simulink model "rtwdemo_sil_hardware_config"  (Simulink 7.6)
settings: Solver=ode3  StartTime=0.0  StopTime=20  FixedStep=0.01  RelTol=1e-3
libraries: rtwdemowidgets x2
Description:
  | Hardware Configuration Options for Software-in-the-Loop Verification
CloseFcn:
  | rtwprivate ssgencode ModelCloseRequest rtwdemo_sil_hardware_config
settings Model: Creator=The MathWorks Inc.  ExtModeAutoUpdateStatusClock=off
settings MATStruct: SampleTime=0.01  Offset=0  Priority=[20.0]
settings DataIOCC: SaveOutput=off  SaveTime=off  SignalLoggingName=sigsOut
settings OptimizationCC: InlineParams=on  InlineInvariantSignals=on  PassReuseOutputArgsAs=Individual arguments  StateBitsets=on  DataBitsets=on  UseTempVars=on  ZeroExternalMemoryAtStartup=off  ZeroInternalMemoryAtStartup=off  NoFixptDivByZeroProtection=on  EfficientFloat2IntCast=on  EfficientMapNaN2IntZero=off  OptimizeModelRefInitCode=on  LifeSpan=1
settings DebuggingCC: UnderspecifiedInitializationDetection=Simplified  MergeDetectMultiDrivingBlocksExec=error  CheckExecutionContextPreStartOutputMsg=on  CheckExecutionContextRuntimeOutputMsg=on  SolverPrmCheckMsg=none  StrictBusMsg=ErrorOnBusTreatedAsVector
settings HardwareCC: ProdBitPerInt=16  ProdIntDivRoundTo=Zero  ProdEndianess=LittleEndian  ProdWordSize=16  ProdHWDeviceType=Generic->16-bit Embedded Processor  TargetEndianess=LittleEndian  TargetHWDeviceType=Generic->MATLAB Host Computer  ProdEqTarget=off
settings RTWCC: SystemTargetFile=ert.tlc  TemplateMakefile=ert_default_tmf  GenerateReport=on  RTWVerbose=off  ProcessScript=ert_make_rtw_hook  IncludeHyperlinkInReport=on  LaunchReport=on
settings CodeAppCC: ForceParamTrailComments=on  IgnoreCustomStorageClasses=off  IgnoreTestpoints=on  SimulinkDataObjDesc=on  CustomSymbolStrGlobalVar=rt$N$M  CustomSymbolStrType=$N$M  CustomSymbolStrFcn=$N$M$F  CustomSymbolStrMacro=$N$M  InsertBlockDesc=on
settings ERTTargetCC: TargetFcnLib=ansi_tfl_tmw.mat  MultiwordLength=2048  GenerateSampleERTMain=on  IncludeMdlTerminateFcn=off  SupportNonFinite=off  SupportComplex=off  SupportContinuousTime=on  GenerateErtSFunction=on  CreateSILPILBlock=SIL  InlinedParameterPlacement=NonHierarchical  ERTCustomFileTemplate=example_file_process.tlc  ERTFilePackagingFormat=CompactWithDataFile  ConvertIfToSwitch=off

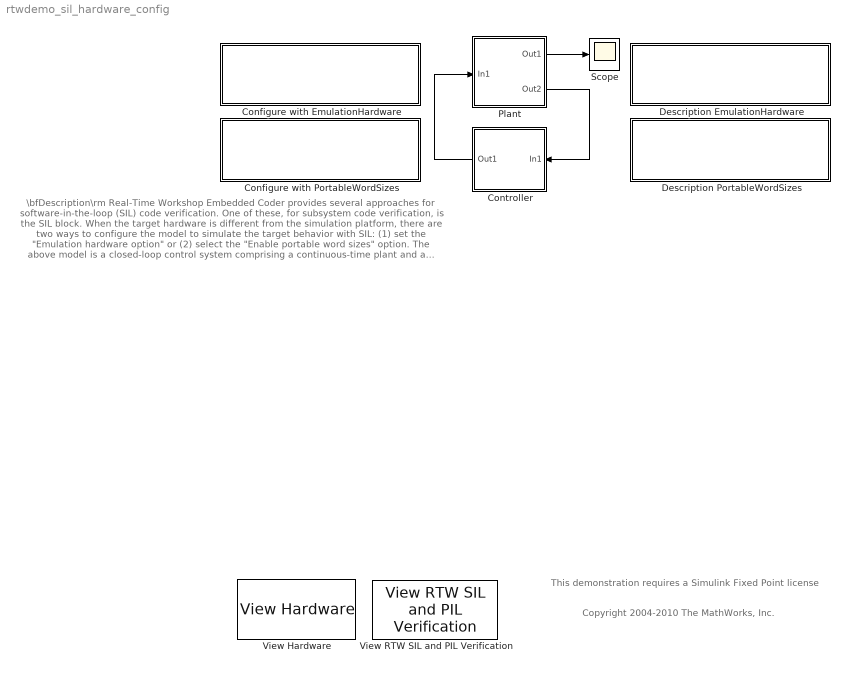
== system rtwdemo_sil_hardware_config ==
  note: \bfDescription\rm
      | Real-Time Workshop Embedded Coder provides several approaches for software-in-the-loop (SIL)
      | code verification. One of these, for subsystem code verification, is the SIL block.
      | When the target hardware is different from the simulation platform, there are two ways to configure
      | the model to simulate the target behavior with SIL: (1) set the "Emulation hardware option" or
      | (2) select the "Enable portable word sizes" option. The above model is a closed-loop control
      | system comprising a continuous-time plant and a discrete-time controller to be deployed on a
      | generic 16-bit microcontroller. The Controller subsystem employs fixed-point arithmetic. An
      | overflow effect is intentionally added to help compare simulation results. To read more about
      | each option, click the above grey buttons. Click the yellow buttons to view the configuration panels.
      |
      | \bfInstructions\rm
      | 1. Click either of the blue buttons above to configure the model automatically.
      | 2. Right-click the Controller subsystem and select Real-Time Workshop > Build Subsystem.
      | 3. When the parameter dialog appears, click the Build button. The SIL block is created in
      |     an untitled model.  This SIL block is an S-function wrapper for the generated subsystem code,
      |     and can be used to verify that the code provides the same result as the original subsystem.
      | 4. Replace the original system with the S-function block and rerun the simulation to verify that the
      |     output is correct. Observe the overflow effect at around 10.8 seconds.
  note: Copyright 2004-2010 The MathWorks, Inc.
  note: This demonstration requires a Simulink Fixed Point license
  Configure with EmulationHardware : Subsystem
      settings: OpenFcn=|
      | try
      |   set_param(gcs, 'GenerateErtSFunction', 'on');
      |   set_param(gcs, 'ProdEqTarget','off');            set_param(gcs, 'PortableWordSizes','off');
      |   set_param(gcs, 'TargetHWDeviceType', 'MATLAB Host');
      | catch
      |   disp('cannot auto configure.');
      |   rethrow(lasterror);
      | end
      mask Type: Auto Config
      mask Display: disp(['Configure with \nEmulation Hardware Setup\n(double-click)'])
  Configure with PortableWordSizes : Subsystem
      settings: OpenFcn=|
      | try
      |   set_param(gcs, 'GenerateErtSFunction', 'on');
      |   set_param(gcs, 'ProdEqTarget','on');             set_param(gcs, 'PortableWordSizes','on');
      | catch
      |     error('cannot auto configure.');
      | end
      mask Display: disp(['Configure with \nPortable Word Sizes Setup\n(double-click)'])
  Controller : Subsystem  TreatAsAtomicUnit=on
      settings: RTWFcnNameOpts=Use subsystem name  RTWFileNameOpts=Use function name
  Description EmulationHardware : Subsystem
      mask Display: disp(['View Description of\n Emulation Hardware Setup\n(double-click)'])
  Description PortableWordSizes : Subsystem
      mask Display: disp(['View Description of \nPortable Word Sizes Setup\n(double-click)'])
  Plant : Subsystem
  Scope : Scope
      settings: TimeRange=20  YMin=0  YMax=400
  View Hardware : rtwdemowidgets/View Hardware  SystemSampleTime=-1
  View RTW SIL and PIL Verification : rtwdemowidgets/View RTW SIL and PIL Verification  SystemSampleTime=-1
  wires:
  Plant/1(Out1) -> Scope/1
  Plant/2(Out2) -> Controller/1(In1)
  Controller/1(Out1) -> Plant/1(In1)

== system rtwdemo_sil_hardware_config/Configure with EmulationHardware ==

== system rtwdemo_sil_hardware_config/Configure with PortableWordSizes ==

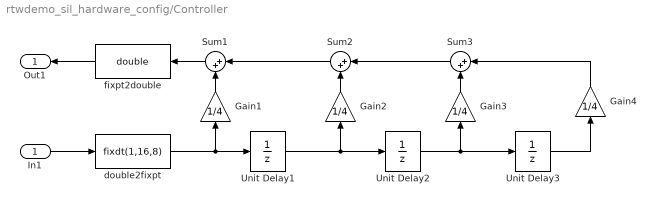
== system rtwdemo_sil_hardware_config/Controller ==
  In1 : Inport  SampleTime=.01
  Gain{1..4} (4 alike) : Gain  Gain=1/4  SaturateOnIntegerOverflow=on  ParamDataTypeStr=Inherit: Same as input
  Sum1 : Sum  Inputs=|++  SaturateOnIntegerOverflow=on  InputSameDT=on  OutDataTypeStr=Inherit: Same as first input
  Sum2 : Sum  Inputs=|++  SaturateOnIntegerOverflow=on  InputSameDT=on  OutDataTypeStr=Inherit: Same as first input
  Sum3 : Sum  Inputs=|++  SaturateOnIntegerOverflow=on  InputSameDT=on  OutDataTypeStr=Inherit: Same as first input
  Unit Delay1 : UnitDelay  SampleTime=-1
  Unit Delay2 : UnitDelay  SampleTime=-1
  Unit Delay3 : UnitDelay  SampleTime=-1
  double2fixpt : DataTypeConversion  OutDataTypeStr=fixdt(1,16,8)
  fixpt2double : DataTypeConversion  OutDataTypeStr=double
  Out1 : Outport
  wires:
  Gain1/1 -> Sum1/2
  In1/1 -> double2fixpt/1
  Sum1/1 -> fixpt2double/1
  Sum3/1 -> Sum2/1
  Sum2/1 -> Sum1/1
  Unit Delay1/1 -> Unit Delay2/1, Gain2/1
  Unit Delay2/1 -> Unit Delay3/1, Gain3/1
  Unit Delay3/1 -> Gain4/1
  Gain4/1 -> Sum3/1
  Gain3/1 -> Sum3/2
  Gain2/1 -> Sum2/2
  double2fixpt/1 -> Unit Delay1/1, Gain1/1
  fixpt2double/1 -> Out1/1

== system rtwdemo_sil_hardware_config/Description EmulationHardware ==
  note: \bfDescription\rm
      | You may need to use the host platform to simulate the exact behavior of the generated code on the
      | embedded system where it will be deployed. Choose to create a SIL block with
      | the emulation hardware set to the host platform.  In this case, Real-Time Workshop inserts any additional
      | code (e.g., data type casts) that is necessary to ensure behavior consistent with the target environment.
      | After the simulation, choose "None" for emulation hardware and regenerate the code before deployment.
      |
      | \bfManual Configuration\rm
      | 1. Open the Hardware Implementation page by double-clicking the first yellow button at the bottom. Select
      |     "MATLAB Host Computer" as Emulation hardware.
      | 2. Open the Real-Time Workshop SIL and PIL Verification page by double-clicking the second yellow
      |      button at the bottom. Ensure that the "Create block" option is set to "SIL" and the
      |     "Enable portable word sizes" option is NOT selected.
      | 3. Apply the changes.

== system rtwdemo_sil_hardware_config/Description PortableWordSizes ==
  note: \bfDescription\rm
      | Often the subsystem to be verified contains algorithms targeted at an embedded system that uses a
      | different word size definition than the host platform. By choosing to create a SIL block with the
      | "Enable portable word sizes" option selected, exact production code to be deployed on the target
      | system is generated then compiled as a Simulink S-function using host platform word size definition.
      |
      | With this option, a preprocessor flag -DPORTABLE\_WORDSIZES can be passed into the compiler to
      | include the host platform based <limit.h> for host-based SIL simulation. After the simulation, the same
      | code can be compiled without the flag to include the actual target <rtwtypes.h> for deployment.
      |
      | \bfManual Configuration\rm
      | 1. Open the Hardware Implementation page by double-clicking the first yellow button at the bottom. Ensure
      |     the "None" checkbox in the Emulation hardware group is selected.
      | 2. Open the Real-Time Workshop SIL and PIL Verification page by double-clicking the second yellow
      |     button at the bottom. Ensure that the "Create block" option is set to "SIL" and the
      |    "Enable portable word sizes" option is selected.
      | 3. Apply the changes.
      |
      | \bfNotes\rm
      | With this method, the numerical results of the S-Function simulation may differ from that of the actual
      | target due to differences in target characteristics such as integral promotion, signed integer division,
      | and signed integer shift right behaviors. See the Real-Time Workshop Embedded Coder documentation for
      | details.

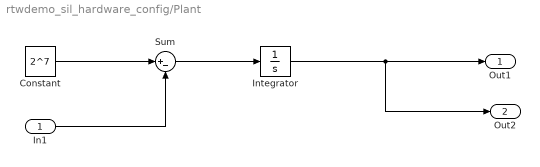
== system rtwdemo_sil_hardware_config/Plant ==
  In1 : Inport
  Constant : Constant  Value=2^7
  Integrator : Integrator
  Sum : Sum  Inputs=|+-  SaturateOnIntegerOverflow=on  InputSameDT=on  OutDataTypeStr=Inherit: Same as first input
  Out1 : Outport
  Out2 : Outport  Port=2
  wires:
  Integrator/1 -> Out1/1, Out2/1
  Sum/1 -> Integrator/1
  Constant/1 -> Sum/1
  In1/1 -> Sum/2
